simulink model "SimpleConveyorSystem"  (R2025b)
settings: Solver=VariableStepAuto  StartTime=0.0  StopTime=1  RelTol=1e-3
settings Model: Creator=KoayXianCong  LastModifiedBy=KoayXianCong
settings ConfigComp: PLC_TargetIDE=gxworks3  PLC_GenerateTestbench=on  PLC_MultiTBSigbuilderTimeRange=off  PLC_FoldFBCallOutputVar=off  PLC_RemoveUnusedSSMethodCallArguments=off  PLC_UseCallOutputArgSyntax=off  PLC_EnableUnsignedAndDoubleTypes=off  PLC_EnableUDTSplitting=off  PLC_MaxFieldsInUDT=500.0  PLC_InlineEnumCastFunction=off  PLC_RTWMaxIdLength=31.0  PLC_RollThreshold=5.0  PLC_ActiveTab=0.0  PLC_EnableStringLiteralTB=on  PLC_Enable64bitIntSupport=off

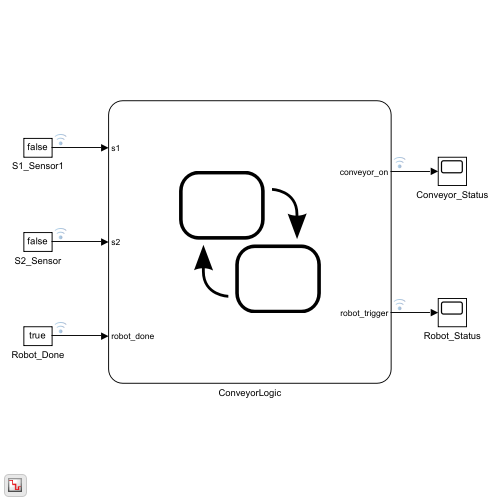
[thumbnail: Simulink's stored preview of the top-level diagram]
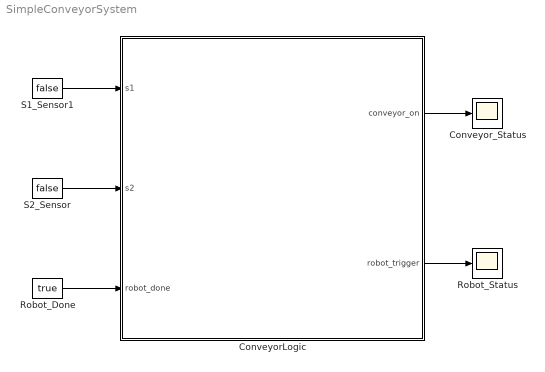
== system SimpleConveyorSystem ==
  ConveyorLogic : Stateflow chart  TreatAsAtomicUnit=on
  Conveyor_Status : Scope
      settings: ActiveDisplayYMinimum=-1  ActiveDisplayYMaximum=1
  Robot_Done : Constant  Value=true  OutDataTypeStr=boolean
  Robot_Status : Scope
      settings: ActiveDisplayYMinimum=-1  ActiveDisplayYMaximum=1
  S1_Sensor1 : Constant  Value=false  OutDataTypeStr=boolean
  S2_Sensor : Constant  Value=false  OutDataTypeStr=boolean
  wires:
  S1_Sensor1/1 -> ConveyorLogic/1(s1)
  Robot_Done/1 -> ConveyorLogic/3(robot_done)
  S2_Sensor/1 -> ConveyorLogic/2(s2)
  ConveyorLogic/1(conveyor_on) -> Conveyor_Status/1
  ConveyorLogic/2(robot_trigger) -> Robot_Status/1

== stateflow chart SimpleConveyorSystem/ConveyorLogic ==
  settings: updateMethod=DISCRETE  sampleTime=0.5
  state IDLE
    entry: conveyor_on = false; robot_trigger = false;
  state MOVING
    during: conveyor_on = true;
  state ROBOT_WORKING
    entry: conveyor_on = false; robot_trigger = true;
    during: conveyor_on = false;
  ROBOT_WORKING -> IDLE : [robot_done && ~s2]
  (default) -> IDLE
  IDLE -> MOVING : [s1 && ~s2]
  MOVING -> ROBOT_WORKING : [s2]
  data: s1 input boolean; s2 input boolean; robot_done input boolean; conveyor_on output boolean; robot_trigger output boolean
